simulink model "CD_Pra6_simulink"  (R2024b)
settings: Solver=VariableStepAuto  StartTime=0.0  StopTime=0.01  RelTol=1e-3
values from neighbouring files (symbols this model uses):
  C = 10e-6    (= 1e-05)    [CD.m]    (also in CD_Valores.m)
  d = 0.385    [CD.m]    (also in CD_Valores.m)
  L = 2e-3    (= 0.002)    [CD.m]    (also in CD_Valores.m)
  R = 10    [CD.m]    (also in CD_Valores.m)
  Ui = 32    [CD.m]    (also in CD_Valores.m)

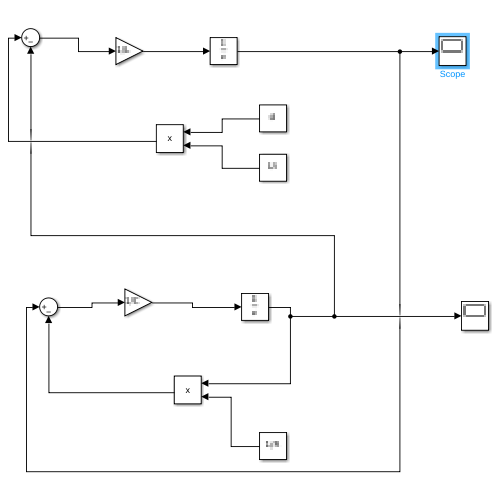
[thumbnail: Simulink's stored preview of the top-level diagram]
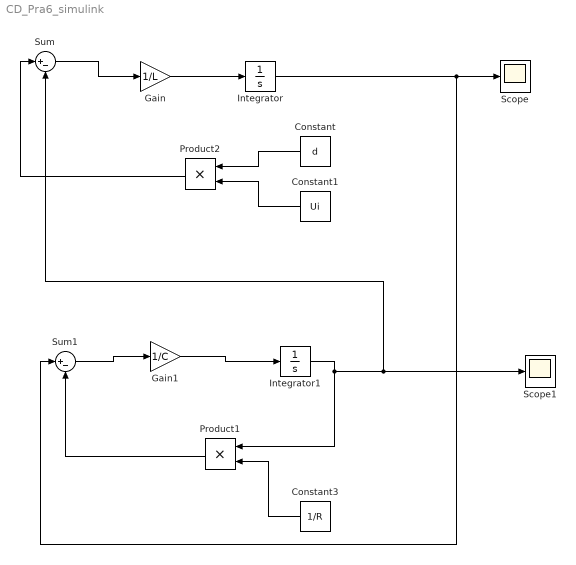
== system CD_Pra6_simulink ==
  Constant : Constant  Value=d
  Constant1 : Constant  Value=Ui
  Constant3 : Constant  Value=1/R
  Gain : Gain  Gain=1/L
  Gain1 : Gain  Gain=1/C
  Integrator : Integrator
  Integrator1 : Integrator
  Product1 : Product
  Product2 : Product
  Scope : Scope
  Scope1 : Scope
  Sum : Sum  Inputs=|+-
  Sum1 : Sum  Inputs=|+-
  wires:
  Constant/1 -> Product2/1
  Constant1/1 -> Product2/2
  Gain/1 -> Integrator/1
  Integrator/1 -> Sum1/1, Scope/1
  Sum/1 -> Gain/1
  Gain1/1 -> Integrator1/1
  Sum1/1 -> Gain1/1
  Product1/1 -> Sum1/2
  Constant3/1 -> Product1/2
  Integrator1/1 -> Sum/2, Scope1/1, Product1/1
  Product2/1 -> Sum/1
